simulink model "sender1"  (R2025a)
settings: Solver=FixedStepAuto  StartTime=0.0  StopTime=10.0  RelTol=1e-3
undefined symbols (not defined in the file): P
libraries: androidsensorlib x2, dspxfrm3 x2, androidaudiovideolib x1, androidcommunicationlib x1
settings Model: Creator=Student  LastModifiedBy=sahas
settings OptimizationCC: DefaultParameterBehavior=Inlined  EnhancedBackFolding=on  PassReuseOutputArgsAs=Individual arguments  ZeroExternalMemoryAtStartup=off  ZeroInternalMemoryAtStartup=off  MaxStackSize=64  OptimizeBlockOrder=speed  DifferentSizesBufferReuse=on  OptimizationCustomize=off  EfficientTunableParamExpr=on
settings DebuggingCC: ParameterTunabilityLossMsg=error
settings HardwareCC: ProdBitPerLong=64.0  ProdLargestAtomicInteger=LongLong  ProdLargestAtomicFloat=Double  ProdLongLongMode=on  ProdHWDeviceType=ARM Compatible->ARM Cortex-A (64-bit)  UseEmbeddedCoderFeatures=off
settings SFSimCC: MATLABDynamicMemAlloc=off
settings RTWCC: SystemTargetFile=ert.tlc  HardwareBoard=Android Device (64bit)  TLCOptions="-aInlineSetEventsForThisBaseRateFcn=TLC_FALSE -aSuppressMultiTaskScheduler=TLC_FALSE  -aRateBasedStepFcn=0"  TemplateMakefile=ert_default_tmf  RTWVerbose=off  Toolchain=Android SDK/NDK Tools  Description=Embedded Coder
settings CodeAppCC: ForceParamTrailComments=on  IgnoreCustomStorageClasses=off  OperatorAnnotations=on  SimulinkDataObjDesc=on  SFDataObjDesc=on  InsertBlockDesc=on
settings ERTTargetCC: ExtModeTransport=0.0  ExtModeStaticAlloc=off  ExtModeMexFile=ext_comm  ExtModeIntrfLevel=Level1  SupportNonInlinedSFcns=on

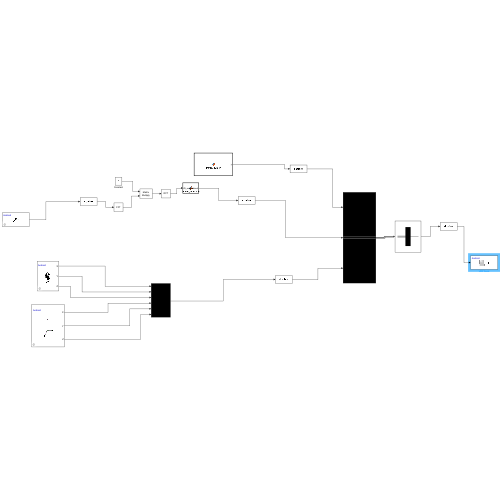
[thumbnail: Simulink's stored preview of the top-level diagram]
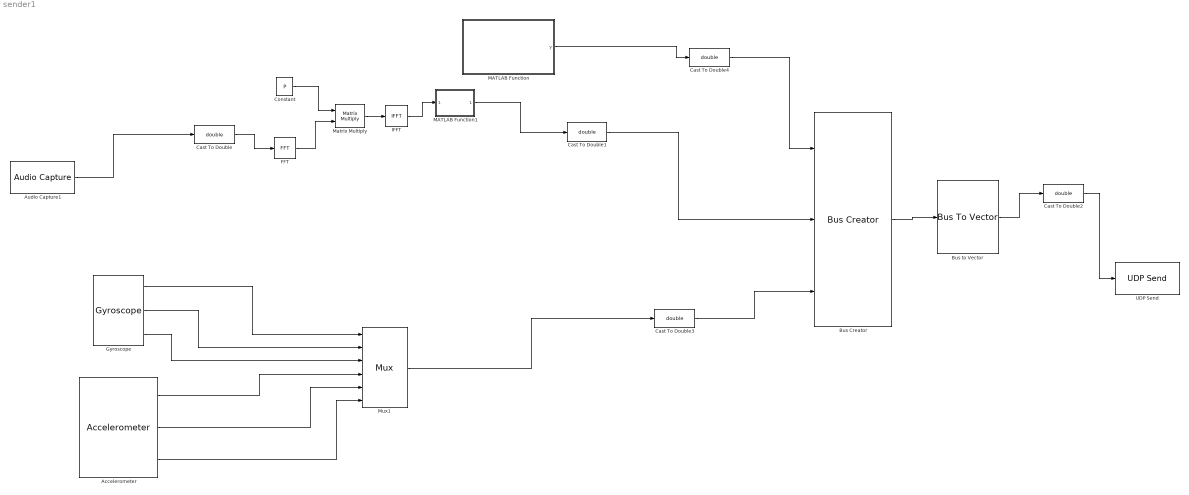
== system sender1 ==
  Accelerometer : androidsensorlib/Accelerometer  OutputVector=off  SampleTime=0.016  BlockPlatform=Android
  Audio Capture1 : androidaudiovideolib/Audio Capture  SampleFreq=16000  FrameSize=256  SampleTime=0.016  SimulateUsing=Code generation  DeviceStr=0  QueueDuration=0  BlockPlatform=Android  AudioSamplingFreq=44100
  Bus Creator : BusCreator  Inputs=3
  Bus to Vector : BusToVector
  Cast To Double{,1..4} (5 alike) : DataTypeConversion  OutDataTypeStr=double  SaturateOnIntegerOverflow=off  RndMeth=Floor
  Constant : Constant  Value=P  VectorParams1D=off
  FFT : dspxfrm3/FFT  FFTImplementation=Auto  CompMethod=Table lookup  TableOpt=NEW  TableOptActive=Speed  BitRevOrder=off  Normalize=off  InheritFFTLength=on  FFTLength=64  WrapInput=on  roundingMode=Ceiling  overflowMode=off  firstCoeffDataTypeStr=Inherit: Same word length as input  firstCoeffLastDataTypeStr=Inherit: Same word length as input  outputMin=[]  outputMax=[]
  Gyroscope : androidsensorlib/Gyroscope  OutputVector=off  SampleTime=0.016  BlockPlatform=Android
  IFFT : dspxfrm3/IFFT  FFTImplementation=Auto  CompMethod=Table lookup  TableOpt=NEW  TableOptActive=Speed  BitRevOrder=off  cs_in=off  Normalize=on  InheritFFTLength=on  FFTLength=64  WrapInput=on  mode=Real  outSamplingMode=Sample based  roundingMode=Ceiling  overflowMode=off  firstCoeffDataTypeStr=Inherit: Same word length as input  firstCoeffLastDataTypeStr=Inherit: Same word length as input  outputMin=[]  outputMax=[]
  MATLAB Function : MATLAB Function  TreatAsAtomicUnit=on
  MATLAB Function1 : MATLAB Function  TreatAsAtomicUnit=on
  Matrix Multiply : Product  Multiplication=Matrix(*)
  Mux1 : Mux  Inputs=6
  UDP Send : androidcommunicationlib/UDP Send  remoteURL='10.7.7.66'  remotePort=28000  localURL='0.0.0.0'  localPortSource=Automatically determine  localPort=-1  sampletime=-1  blockPlatform=Android  separateLengthPort=0
  wires:
  Constant/1 -> Matrix Multiply/1
  Matrix Multiply/1 -> IFFT/1
  FFT/1 -> Matrix Multiply/2
  Cast To Double/1 -> FFT/1
  Audio Capture1/1 -> Cast To Double/1
  IFFT/1 -> MATLAB Function1/1(ifft_output)
  MATLAB Function1/1(combined) -> Cast To Double1/1
  Cast To Double2/1 -> UDP Send/1
  Mux1/1 -> Cast To Double3/1
  Cast To Double1/1 -> Bus Creator/2
  Bus Creator/1 -> Bus to Vector/1
  Bus to Vector/1 -> Cast To Double2/1
  MATLAB Function/1(y) -> Cast To Double4/1
  Cast To Double3/1 -> Bus Creator/3
  Cast To Double4/1 -> Bus Creator/1
  Gyroscope/1 -> Mux1/1
  Gyroscope/2 -> Mux1/2
  Gyroscope/3 -> Mux1/3
  Accelerometer/1 -> Mux1/4
  Accelerometer/2 -> Mux1/5
  Accelerometer/3 -> Mux1/6

== matlab function sender1/MATLAB Function ==
  data: y output
function y = frameCounter()
persistent n
if isempty(n), n = 0; end
n = n + 1;
y = n;
end

== matlab function sender1/MATLAB Function1 ==
  data: ifft_output input; combined output
function combined = sender_interleave(ifft_output)
%#codegen

% Split real and imaginary parts
real_part = real(ifft_output);  % 512x2
imag_part = imag(ifft_output);  % 512x2

% Flatten column-wise
real_flat = real_part(:);  % 1024x1
imag_flat = imag_part(:);  % 1024x1

% Interleave into 1-D array: [real1 imag1 real2 imag2 ...]
combined = zeros(2*numel(real_flat),1);
combined(1:2:end) = real_flat;
combined(2:2:end) = imag_flat;


end
